simulink model "p1"  (R2021b)
settings: Solver=VariableStepAuto  StartTime=0.0  StopTime=0.1  RelTol=1e-3
values from neighbouring files (symbols this model uses):
  a = 20*pi/180    (= 0.349065850399)    [P1_Concentrated_mass_method.m]    (also in P1_odefun.m)
  c1 = 900    [P1_Concentrated_mass_method.m]    (also in P1_odefun.m)
  c2 = 900    [P1_Concentrated_mass_method.m]    (also in P1_odefun.m)
  cm = 1000    [P1_Concentrated_mass_method.m]
  g = 9.8    [P1_Concentrated_mass_method.m]    (also in P1_odefun.m)
  I1 = 0.0033    [P1_Concentrated_mass_method.m]    (also in P1_odefun.m)
  I2 = 0.0115    [P1_Concentrated_mass_method.m]    (also in P1_odefun.m)
  k1 = 2*1e8    (= 200000000)    [P1_Concentrated_mass_method.m]    (also in P1_odefun.m)
  k2 = 2*1e8    (= 200000000)    [P1_Concentrated_mass_method.m]    (also in P1_odefun.m)
  km = 1*1e8    (= 100000000)    [P1_Concentrated_mass_method.m]
  m1 = 2.034    [P1_Concentrated_mass_method.m]    (also in P1_odefun.m)
  m2 = 3.973    [P1_Concentrated_mass_method.m]    (also in P1_odefun.m)
  rb1 = z1*m/2*cos(a)*1e-3    [P1_Concentrated_mass_method.m]    (also in P1_odefun.m)
  rb2 = z2*m/2*cos(a)*1e-3    [P1_Concentrated_mass_method.m]    (also in P1_odefun.m)
  T1 = 31.9    [P1_Concentrated_mass_method.m]    (also in P1_odefun.m)
  T2 = 68.8    [P1_Concentrated_mass_method.m]    (also in P1_odefun.m)
settings Model: Creator=11639  LastModifiedBy=11639

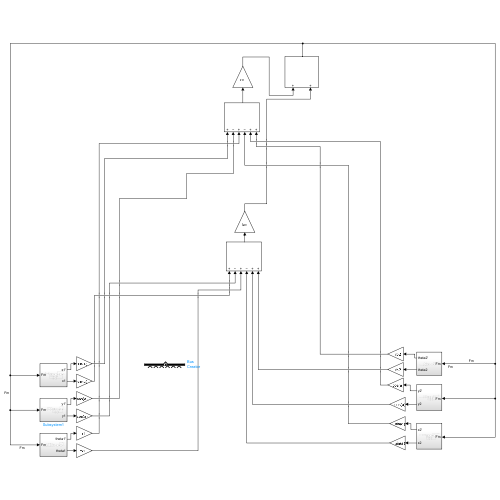
[thumbnail: Simulink's stored preview of the top-level diagram]
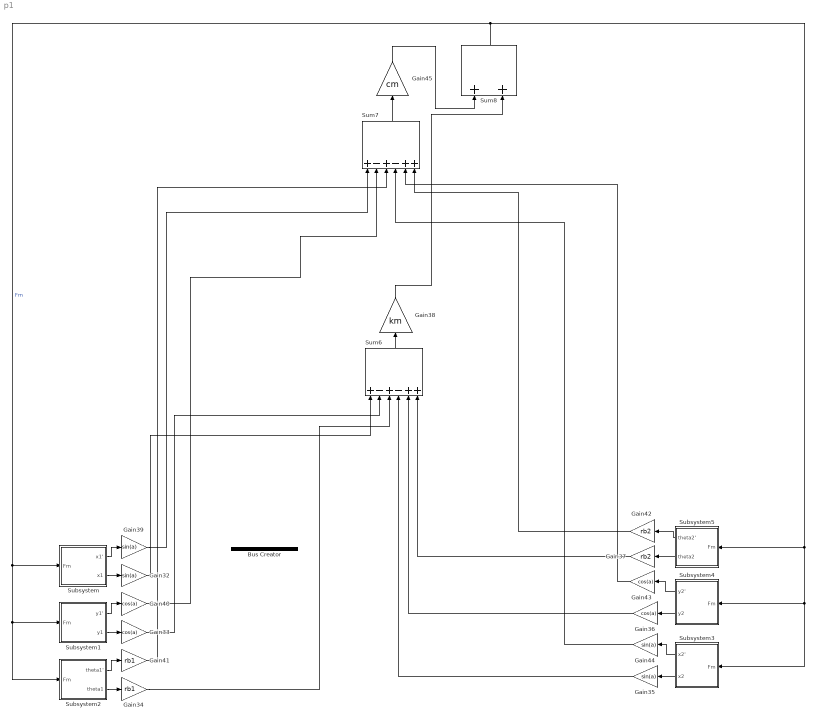
== system p1 ==
  Bus Creator : BusCreator  Inputs=6
  Gain{32,35,39,44} (4 alike) : Gain  Gain=sin(a)
  Gain{33,36,40,43} (4 alike) : Gain  Gain=cos(a)
  Gain34 : Gain  Gain=rb1
  Gain37 : Gain  Gain=rb2
  Gain38 : Gain  Gain=km
  Gain41 : Gain  Gain=rb1
  Gain42 : Gain  Gain=rb2
  Gain45 : Gain  Gain=cm
  Subsystem : Subsystem
  Subsystem1 : Subsystem
  Subsystem2 : Subsystem
  Subsystem3 : Subsystem
  Subsystem4 : Subsystem
  Subsystem5 : Subsystem
  Sum6 : Sum  Inputs=+-+-++
  Sum7 : Sum  Inputs=+-+-++
  Sum8 : Sum
  wires:
  Sum8/1 -> Subsystem5/1(Fm), Subsystem4/1(Fm), Subsystem3/1(Fm), Subsystem2/1(Fm), Subsystem1/1(Fm), Subsystem/1(Fm)  "Fm"
  Gain32/1 -> Sum6/1
  Gain33/1 -> Sum6/2
  Gain34/1 -> Sum6/3
  Gain35/1 -> Sum6/4
  Gain36/1 -> Sum6/5
  Gain37/1 -> Sum6/6
  Sum6/1 -> Gain38/1
  Gain39/1 -> Sum7/1
  Gain40/1 -> Sum7/2
  Gain41/1 -> Sum7/3
  Gain44/1 -> Sum7/4
  Gain43/1 -> Sum7/5
  Gain42/1 -> Sum7/6
  Sum7/1 -> Gain45/1
  Gain45/1 -> Sum8/1
  Gain38/1 -> Sum8/2
  Subsystem/2(x1) -> Gain32/1
  Subsystem/1(x1') -> Gain39/1
  Subsystem1/2(y1) -> Gain33/1
  Subsystem1/1(y1') -> Gain40/1
  Subsystem2/2(theta1) -> Gain34/1
  Subsystem2/1(theta1') -> Gain41/1
  Subsystem3/2(x2) -> Gain35/1
  Subsystem3/1(x2') -> Gain44/1
  Subsystem4/2(y2) -> Gain36/1
  Subsystem4/1(y2') -> Gain43/1
  Subsystem5/2(theta2) -> Gain37/1
  Subsystem5/1(theta2') -> Gain42/1

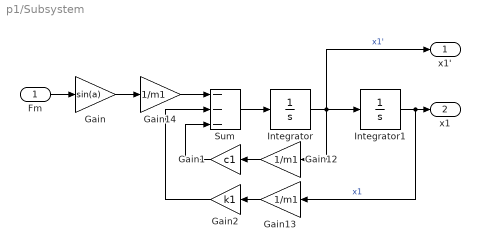
== system p1/Subsystem ==
  Fm : Inport
  Gain : Gain  Gain=sin(a)
  Gain1 : Gain  Gain=c1
  Gain12 : Gain  Gain=1/m1
  Gain13 : Gain  Gain=1/m1
  Gain14 : Gain  Gain=1/m1
  Gain2 : Gain  Gain=k1
  Integrator : Integrator
  Integrator1 : Integrator
  Sum : Sum  Inputs=---
  x1' : Outport
  x1 : Outport  Port=2
  wires:
  Gain1/1 -> Sum/3
  Gain2/1 -> Sum/2
  Gain12/1 -> Gain1/1
  Gain/1 -> Gain14/1
  Gain13/1 -> Gain2/1
  Sum/1 -> Integrator/1
  Integrator/1 -> x1'/1, Gain12/1, Integrator1/1  "x1'"
  Gain14/1 -> Sum/1
  Integrator1/1 -> Gain13/1, x1/1  "x1"
  Fm/1 -> Gain/1

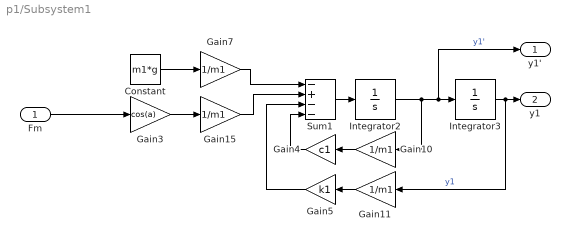
== system p1/Subsystem1 ==
  Fm : Inport
  Constant : Constant  Value=m1*g
  Gain{7,10..11,15} (4 alike) : Gain  Gain=1/m1
  Gain3 : Gain  Gain=cos(a)
  Gain4 : Gain  Gain=c1
  Gain5 : Gain  Gain=k1
  Integrator2 : Integrator
  Integrator3 : Integrator
  Sum1 : Sum  Inputs=-+--
  y1' : Outport
  y1 : Outport  Port=2
  wires:
  Integrator2/1 -> y1'/1, Integrator3/1, Gain10/1  "y1'"
  Fm/1 -> Gain3/1
  Sum1/1 -> Integrator2/1
  Gain10/1 -> Gain4/1
  Gain7/1 -> Sum1/1
  Gain5/1 -> Sum1/3
  Constant/1 -> Gain7/1
  Gain4/1 -> Sum1/4
  Gain3/1 -> Gain15/1
  Gain11/1 -> Gain5/1
  Gain15/1 -> Sum1/2
  Integrator3/1 -> Gain11/1, y1/1  "y1"

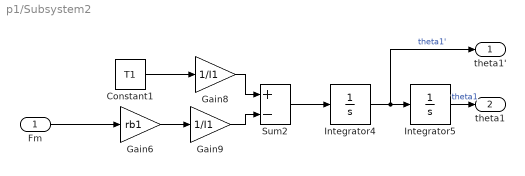
== system p1/Subsystem2 ==
  Fm : Inport
  Constant1 : Constant  Value=T1
  Gain6 : Gain  Gain=rb1
  Gain8 : Gain  Gain=1/I1
  Gain9 : Gain  Gain=1/I1
  Integrator4 : Integrator
  Integrator5 : Integrator
  Sum2 : Sum  Inputs=+-
  theta1' : Outport
  theta1 : Outport  Port=2
  wires:
  Integrator4/1 -> theta1'/1, Integrator5/1  "theta1'"
  Gain6/1 -> Gain9/1
  Gain9/1 -> Sum2/2
  Sum2/1 -> Integrator4/1
  Constant1/1 -> Gain8/1
  Gain8/1 -> Sum2/1
  Fm/1 -> Gain6/1
  Integrator5/1 -> theta1/1  "theta1"

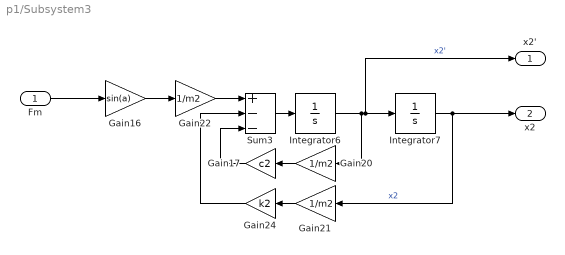
== system p1/Subsystem3 ==
  Fm : Inport
  Gain16 : Gain  Gain=sin(a)
  Gain17 : Gain  Gain=c2
  Gain20 : Gain  Gain=1/m2
  Gain21 : Gain  Gain=1/m2
  Gain22 : Gain  Gain=1/m2
  Gain24 : Gain  Gain=k2
  Integrator6 : Integrator
  Integrator7 : Integrator
  Sum3 : Sum  Inputs=+--
  x2' : Outport
  x2 : Outport  Port=2
  wires:
  Integrator6/1 -> x2'/1, Integrator7/1, Gain20/1  "x2'"
  Gain20/1 -> Gain17/1
  Gain24/1 -> Sum3/2
  Sum3/1 -> Integrator6/1
  Gain22/1 -> Sum3/1
  Integrator7/1 -> x2/1, Gain21/1  "x2"
  Gain17/1 -> Sum3/3
  Gain21/1 -> Gain24/1
  Gain16/1 -> Gain22/1
  Fm/1 -> Gain16/1

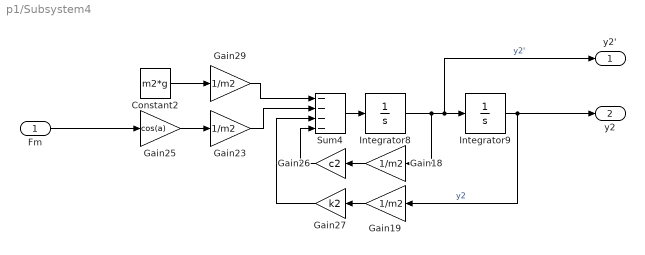
== system p1/Subsystem4 ==
  Fm : Inport
  Constant2 : Constant  Value=m2*g
  Gain{18..19,23,29} (4 alike) : Gain  Gain=1/m2
  Gain25 : Gain  Gain=cos(a)
  Gain26 : Gain  Gain=c2
  Gain27 : Gain  Gain=k2
  Integrator8 : Integrator
  Integrator9 : Integrator
  Sum4 : Sum  Inputs=----
  y2' : Outport
  y2 : Outport  Port=2
  wires:
  Gain19/1 -> Gain27/1
  Gain25/1 -> Gain23/1
  Integrator8/1 -> y2'/1, Integrator9/1, Gain18/1  "y2'"
  Gain23/1 -> Sum4/2
  Gain26/1 -> Sum4/4
  Fm/1 -> Gain25/1
  Constant2/1 -> Gain29/1
  Gain18/1 -> Gain26/1
  Integrator9/1 -> y2/1, Gain19/1  "y2"
  Gain29/1 -> Sum4/1
  Sum4/1 -> Integrator8/1
  Gain27/1 -> Sum4/3

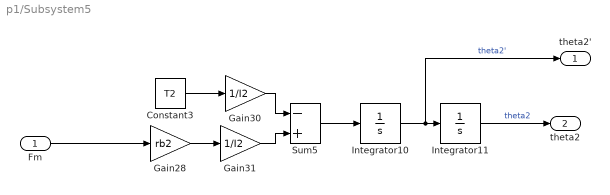
== system p1/Subsystem5 ==
  Fm : Inport
  Constant3 : Constant  Value=T2
  Gain28 : Gain  Gain=rb2
  Gain30 : Gain  Gain=1/I2
  Gain31 : Gain  Gain=1/I2
  Integrator10 : Integrator
  Integrator11 : Integrator
  Sum5 : Sum  Inputs=-+
  theta2' : Outport
  theta2 : Outport  Port=2
  wires:
  Gain31/1 -> Sum5/2
  Fm/1 -> Gain28/1
  Constant3/1 -> Gain30/1
  Gain28/1 -> Gain31/1
  Gain30/1 -> Sum5/1
  Sum5/1 -> Integrator10/1
  Integrator10/1 -> theta2'/1, Integrator11/1  "theta2'"
  Integrator11/1 -> theta2/1  "theta2"
